simulink model "X001_AL5D_Assemby_RR_013"  (R2016a)
settings: Solver=VariableStepAuto  StartTime=0.0  StopTime=2  RelTol=1e-3
model workspace: external: MATLAB File C:\Users\Home\Google Drive\Engineering Design\Year 4 - Specialisations\Design Project 4 - Systems for Independent Living\Content\MZ\Active_Documents\AL5D Multibody Simulations\X001_AL5D_Assemby_RR_DataFile.m (data not in the file)
values from neighbouring files (symbols this model uses):
  CA = 45    [AL5D_Dataset_Creator.m]
  CAr = degtorad(CA)    [AL5D_Dataset_Creator.m]
  CFTR = CFT+(CFT*perc_disc*normrnd(0,0.5))    [AL5D_Dataset_Creator.m]
  DC = 0.09    [AL5D_Dataset_Creator.m]
  disturbance_time = 0.5    [AL5D_Dataset_Creator.m]
  disturbance_torque = disturbance_torque_array(t)    [AL5D_Dataset_Creator.m]
  DST = 0.2    [AL5D_Dataset_Creator.m]
  first_ref = first_ref_array(f)    [AL5D_Dataset_Creator.m]
  L_0 = l1+l2    (= 0.46066)    [AL5D_Dataset_Creator.m]
  RV1 = 6*2    (= 12)    [AL5D_Dataset_Creator.m]
  SC = (MM*AA)/ML    (= 50)    [AL5D_Dataset_Creator.m]
  second_ref = 0    [AL5D_Dataset_Creator.m]
  second_ref_time = 0    [AL5D_Dataset_Creator.m]
  Ts = 0.0005    [AL5D_Dataset_Creator.m]
  VS = radtodeg(1)    [AL5D_Dataset_Creator.m]
undefined symbols (not defined in the file or in its folder): smiData, X, Y, Z
libraries: sm_lib x33, fl_lib x21, nesl_utility x17, elec_lib x3, dspsrcs4 x2, simulink x1
(part 1 of 2)
settings Model: Creator=Home  LastModifiedBy=Home
settings GRTTargetCC: GeneratePreprocessorConditionals=Use local settings

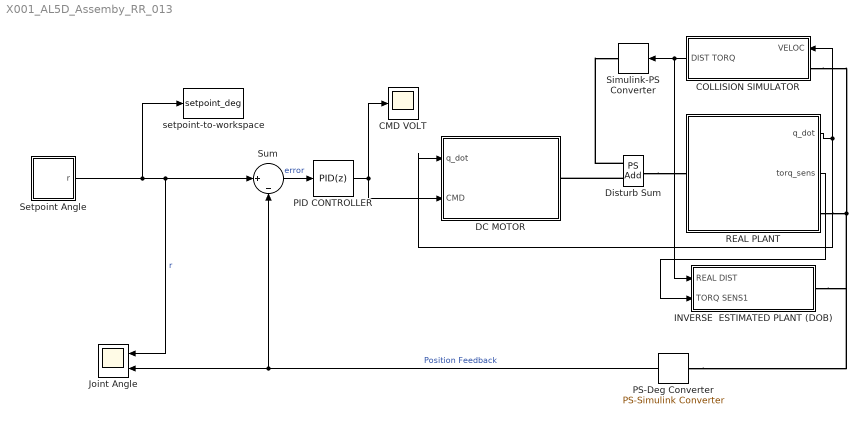
== system X001_AL5D_Assemby_RR_013 ==
  CMD VOLT : Scope
  COLLISION SIMULATOR : Subsystem
  DC MOTOR : Subsystem
  Disturb Sum : fl_lib/Physical Signals/Functions/PS Add
  INVERSE  ESTIMATED PLANT (DOB) : Subsystem
  Joint Angle : Scope  NumInputPorts=2
  PID CONTROLLER : simulink/Continuous/PID Controller  Controller=PID  TimeDomain=Discrete-time  SampleTime=Ts  IntegratorMethod=Forward Euler  FilterMethod=Forward Euler  Form=Parallel  UseFilter=on  ControllerParametersSource=internal  P=8.56066056005533  I=73.9193110956432  D=0.0561082509570558  N=2357.56103079076  InitialConditionSource=internal  InitialConditionForIntegrator=0  InitialConditionForFilter=0  ExternalReset=none  LimitOutput=on  UpperSaturationLimit=RV1  LowerSaturationLimit=-RV1  LinearizeAsGain=off  AntiWindupMode=clamping  Kb=1  TrackingMode=off  Kt=1  PParamMin=[]  PParamMax=[]  IParamMin=[]  IParamMax=[]  DParamMin=[]  DParamMax=[]  NParamMin=[]  NParamMax=[]  KbParamMin=[]  KbParamMax=[]  KtParamMin=[]  KtParamMax=[]  POutMin=[]  POutMax=[]  IOutMin=[]  IOutMax=[]  DOutMin=[]  DOutMax=[]  NOutMin=[]  NOutMax=[]  KbOutMin=[]  KbOutMax=[]  KtOutMin=[]  KtOutMax=[]  IntegratorOutMin=[]  IntegratorOutMax=[]  FilterOutMin=[]  FilterOutMax=[]  SumOutMin=[]  SumOutMax=[]  SumI1OutMin=[]  SumI1OutMax=[]  SumI2OutMin=[]  SumI2OutMax=[]  SumI3OutMin=[]  SumI3OutMax=[]  SumDOutMin=[]  SumDOutMax=[]  SaturationOutMin=[]  SaturationOutMax=[]  IntegratorContinuousStateAttributes=''  IntegratorStateMustResolveToSignalObject=off  IntegratorRTWStateStorageClass=Auto  FilterContinuousStateAttributes=''  FilterStateMustResolveToSignalObject=off  FilterRTWStateStorageClass=Auto  DifferentiatorICPrevScaledInput=0  DifferentiatorOutMin=[]  DifferentiatorOutMax=[]
  PS-Deg Converter : nesl_utility/PS-Simulink Converter  PhysicalDomain=network_engine_domain  SubClassName=ps_output  LeftPortType=input  RightPortType=output  PseudoPeriodic=off  Frequencies=[]  Unit=deg  AffineConversion=off
  REAL PLANT : Subsystem
  Setpoint Angle : Subsystem
  Simulink-PS Converter : nesl_utility/Simulink-PS Converter  PhysicalDomain=network_engine_domain  SubClassName=ps_input  LeftPortType=input  RightPortType=output  PseudoPeriodic=off  Frequencies=[]  NoiseDistribution=none  NoiseParameters=[]  Unit=N*m  AffineConversion=off  InputFiltering=off  SimscapeFilterOrder=1  InputFilterTimeConstant=0.001  UdotUserProvided=1
  Sum : Sum  Inputs=||+|-
  setpoint-to-workspace : ToWorkspace  VariableName=setpoint_deg  SaveFormat=Structure With Time  SampleTime=-1
  wires:
  PID CONTROLLER/1 -> DC MOTOR/2("CMD "), CMD VOLT/1
  Sum/1 -> PID CONTROLLER/1  "error"
  PS-Deg Converter/1 -> Sum/2, Joint Angle/2  "Position Feedback"
  REAL PLANT/1(q_dot) -> DC MOTOR/1(q_dot), COLLISION SIMULATOR/1(VELOC)
  COLLISION SIMULATOR/1(DIST TORQ) -> INVERSE  ESTIMATED PLANT (DOB)/1(REAL DIST), Simulink-PS Converter/1
  Setpoint Angle/1(r) -> setpoint-to-workspace/1, Sum/1, Joint Angle/1  "r"
  REAL PLANT/2(torq_sens) -> INVERSE  ESTIMATED PLANT (DOB)/2(TORQ SENS1)
  connections:
  Disturb Sum/LConn2 -- DC MOTOR/RConn1
  Disturb Sum/RConn1 -- REAL PLANT/LConn1
  REAL PLANT/RConn1 -- PS-Deg Converter/LConn1 -- INVERSE  ESTIMATED PLANT (DOB)/RConn1 -- COLLISION SIMULATOR/LConn1
  Disturb Sum/LConn1 -- Simulink-PS Converter/RConn1

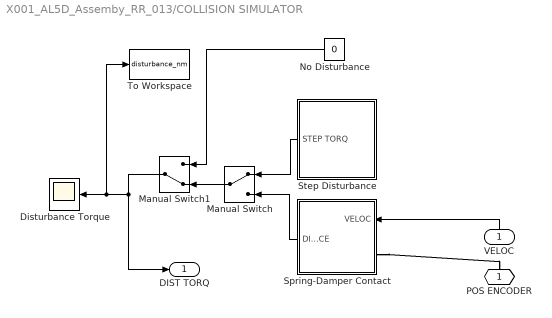
== system X001_AL5D_Assemby_RR_013/COLLISION SIMULATOR ==
  VELOC : Inport
  Disturbance Torque : Scope
  Manual Switch : ManualSwitch
  Manual Switch1 : ManualSwitch  CurrentSetting=0
  No Disturbance : Constant  Value=0
  Spring-Damper Contact : Subsystem
  Step Disturbance : Subsystem
  To Workspace : ToWorkspace  VariableName=disturbance_nm  SaveFormat=Structure With Time  SampleTime=-1
  POS ENCODER : PMIOPort  Port=1  Side=Left
  DIST TORQ : Outport
  wires:
  VELOC/1 -> Spring-Damper Contact/1(VELOC)
  Spring-Damper Contact/1(DISTURBANCE) -> Manual Switch/2
  Step Disturbance/1(STEP TORQ) -> Manual Switch/1
  Manual Switch/1 -> Manual Switch1/2
  No Disturbance/1 -> Manual Switch1/1
  Manual Switch1/1 -> To Workspace/1, Disturbance Torque/1, DIST TORQ/1
  connections:
  Spring-Damper Contact/LConn1 -- POS ENCODER/RConn1

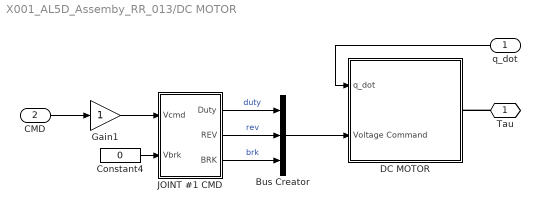
== system X001_AL5D_Assemby_RR_013/DC MOTOR ==
  q_dot : Inport
  "CMD " : Inport  Port=2
  Bus Creator : BusCreator  Inputs=3
  Constant4 : Constant  Value=0  SampleTime=Ts
  DC MOTOR : Subsystem
  Gain1 : Gain
  JOINT #1 CMD : Subsystem
  Tau : PMIOPort  Port=1  Side=Right
  wires:
  JOINT #1 CMD/1(Duty) -> Bus Creator/1  "duty"
  JOINT #1 CMD/2(REV) -> Bus Creator/2  "rev"
  Bus Creator/1 -> DC MOTOR/2(Voltage Command)
  Gain1/1 -> JOINT #1 CMD/1(Vcmd)
  JOINT #1 CMD/3(BRK) -> Bus Creator/3  "brk"
  Constant4/1 -> JOINT #1 CMD/2(Vbrk)
  "CMD "/1 -> Gain1/1
  q_dot/1 -> DC MOTOR/1(q_dot)
  connections:
  Tau/RConn1 -- DC MOTOR/RConn1

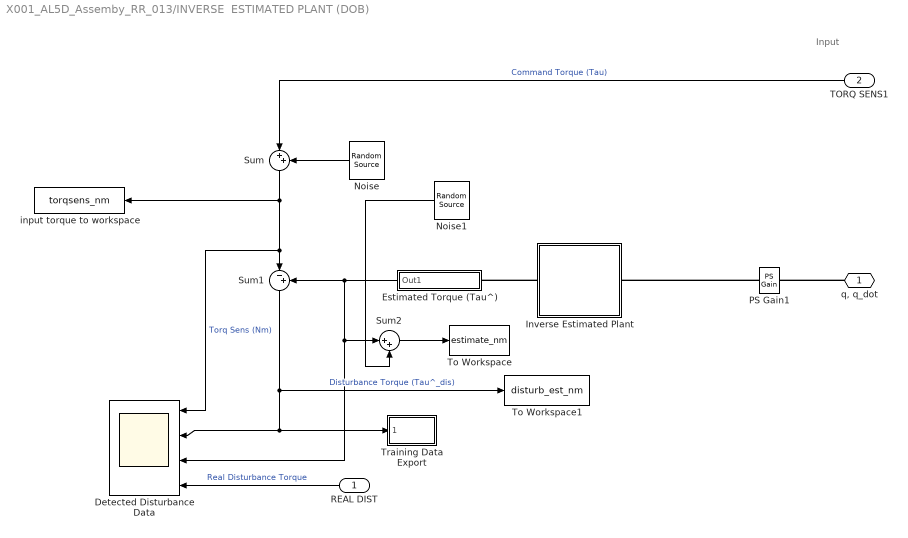
== system X001_AL5D_Assemby_RR_013/INVERSE  ESTIMATED PLANT (DOB) ==
  note: Input
  REAL DIST : Inport
  TORQ SENS1 : Inport  Port=2
  Detected Disturbance Data : Scope  NumInputPorts=4
  Estimated Torque (Tau^) : Subsystem
  Inverse Estimated Plant : Subsystem
  Noise : dspsrcs4/Random Source  SrcType=Uniform  NormMethod=Ziggurat  CltLength=12  MinVal=0  MaxVal=0.1  MeanVal=0  VarVal=1  RepMode=Not repeatable  rawSeed=1  IsInherit=off  SampMode=Discrete  SampTime=Ts*5  SampFrame=1  DataType=Double  OutComplex=Real  OutputFrames=off
  Noise1 : dspsrcs4/Random Source  SrcType=Uniform  NormMethod=Ziggurat  CltLength=12  MinVal=0  MaxVal=0.1  MeanVal=0  VarVal=1  RepMode=Not repeatable  rawSeed=1  IsInherit=off  SampMode=Discrete  SampTime=Ts*5  SampFrame=1  DataType=Double  OutComplex=Real  OutputFrames=off
  PS Gain1 : fl_lib/Physical Signals/Functions/PS Gain  gain=-1
  Sum : Sum  Inputs=|++
  Sum1 : Sum  Inputs=|-+
  Sum2 : Sum  Inputs=|++
  To Workspace : ToWorkspace  VariableName=estimate_nm  SaveFormat=Structure With Time  SampleTime=-1
  To Workspace1 : ToWorkspace  VariableName=disturb_est_nm  SaveFormat=Structure With Time  SampleTime=-1
  Training Data Export : Subsystem
  "input torque to workspace " : ToWorkspace  VariableName=torqsens_nm  SaveFormat=Structure With Time  SampleTime=-1
  "q, q_dot" : PMIOPort  Port=1  Side=Right
  wires:
  REAL DIST/1 -> Detected Disturbance Data/4  "Real Disturbance Torque"
  Sum1/1 -> To Workspace1/1, Detected Disturbance Data/2, Training Data Export/1(tau^_in)  "Disturbance Torque (Tau^_dis)"
  Estimated Torque (Tau^)/1(Out1) -> Sum2/1, Detected Disturbance Data/3, Sum1/2
  Sum/1 -> Detected Disturbance Data/1, Sum1/1, "input torque to workspace "/1  "Torq Sens (Nm)"
  TORQ SENS1/1 -> Sum/1  "Command Torque (Tau)"
  Noise/1 -> Sum/2
  Noise1/1 -> Sum2/2
  Sum2/1 -> To Workspace/1
  connections:
  Inverse Estimated Plant/RConn1 -- Estimated Torque (Tau^)/LConn1
  "q, q_dot"/RConn1 -- PS Gain1/LConn1
  PS Gain1/RConn1 -- Inverse Estimated Plant/LConn1

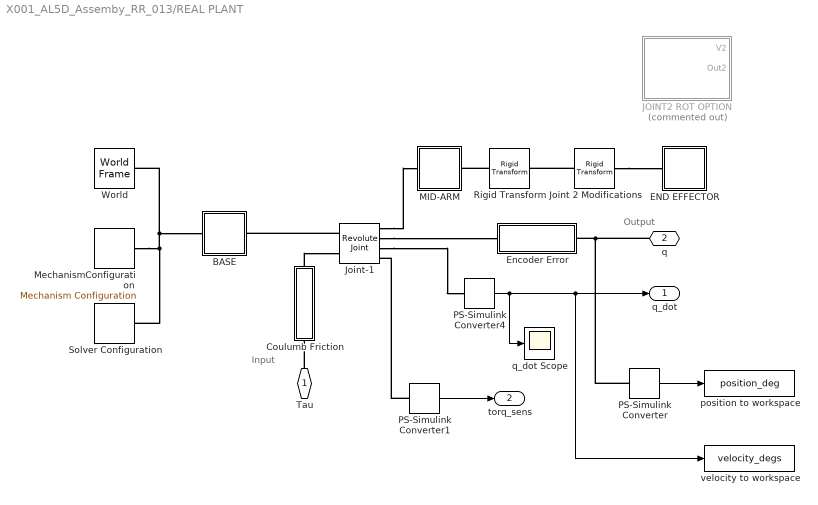
== system X001_AL5D_Assemby_RR_013/REAL PLANT ==
  note: Output
  note: Input
  BASE : Subsystem
  Coulumb Friction : Subsystem
  END EFFECTOR : Subsystem
  Encoder Error : Subsystem
  JOINT2 ROT OPTION : Subsystem  Commented=on
  Joint 2 Modifications : sm_lib/Frames and Transforms/Rigid Transform  TranslationMethod=None  TranslationLengthUnit=m  TranslationStandardAxis=+Z  TranslationStandardOffset=0  TranslationCartesianOffset=[0 0 0]  TranslationROffset=0  TranslationROffsetUnits=m  TranslationZOffset=0  TranslationZOffsetUnits=m  TranslationThetaOffset=0  TranslationThetaOffsetUnits=deg  RotationMethod=StandardAxis  RotationAngleUnits=deg  RotationStandardAxis=+Z  RotationAngle=0  RotationArbitraryAxis=[0 0 1]  FollAlignAxisA=+X  BaseAlignAxisA=+Y  FollAlignAxisB=+Y  BaseAlignAxisB=+Z  RotationSequenceAxes=FollowerAxes  RotationSequence=XYX  RotationSequenceAngles=[0 0 0]  RotationSequenceAnglesUnits=deg  RotationMatrix=[1 0 0; 0 1 0; 0 0 1]
  Joint-1 : sm_lib/Joints/Revolute Joint  SenseConstraintForce=off  SenseConstraintForceX=off  SenseConstraintForceY=off  SenseConstraintForceZ=off  SenseConstraintTorque=off  SenseConstraintTorqueX=off  SenseConstraintTorqueY=off  SenseConstraintTorqueZ=off  SenseTotalForce=off  SenseTotalForceX=off  SenseTotalForceY=off  SenseTotalForceZ=off  SenseTotalTorque=off  SenseTotalTorqueX=off  SenseTotalTorqueY=off  SenseTotalTorqueZ=off  CompositeWrenchDir=FollowerOnBase  CompositeWrenchFrame=BaseFrame  EquilibriumPosition=0  EquilibriumPositionUnits=rad  SpringStiffness=JSSR  SpringStiffnessUnits=m*N/rad  DampingCoefficient=JDCR  DampingCoefficientUnits=m*s*N/rad  TorqueActuationMode=InputTorque  MotionActuationMode=ComputedMotion  SensePosition=on  SenseVelocity=on  SenseAcceleration=off  SenseTorqueForce=on  PositionTargetSpecify=off  PositionTargetPriority=Low  PositionTargetValue=-90  PositionTargetValueUnits=deg  VelocityTargetSpecify=off  VelocityTargetPriority=High  VelocityTargetValue=-30  VelocityTargetValueUnits=deg/s
  MID-ARM : Subsystem
  MechanismConfiguration : sm_lib/Utilities/Mechanism Configuration  UniformGravity=Constant  GravityVector=[0 0 -9.81]  GravityUnits=m/s^2  LinearizationDelta=0.001
  PS-Simulink Converter : nesl_utility/PS-Simulink Converter  PhysicalDomain=network_engine_domain  SubClassName=ps_output  LeftPortType=input  RightPortType=output  PseudoPeriodic=off  Frequencies=[]  Unit=deg  AffineConversion=off
  PS-Simulink Converter1 : nesl_utility/PS-Simulink Converter  PhysicalDomain=network_engine_domain  SubClassName=ps_output  LeftPortType=input  RightPortType=output  PseudoPeriodic=off  Frequencies=[]  Unit=N*m  AffineConversion=off
  PS-Simulink Converter4 : nesl_utility/PS-Simulink Converter  PhysicalDomain=network_engine_domain  SubClassName=ps_output  LeftPortType=input  RightPortType=output  PseudoPeriodic=off  Frequencies=[]  Unit=deg/s  AffineConversion=off
  Rigid Transform : sm_lib/Frames and Transforms/Rigid Transform  TranslationMethod=None  TranslationLengthUnit=m  TranslationStandardAxis=+Z  TranslationStandardOffset=0  TranslationCartesianOffset=[0 0 0]  TranslationROffset=0  TranslationROffsetUnits=m  TranslationZOffset=0  TranslationZOffsetUnits=m  TranslationThetaOffset=0  TranslationThetaOffsetUnits=deg  RotationMethod=ArbitraryAxis  RotationAngleUnits=deg  RotationStandardAxis=+Z  RotationAngle=-90  RotationArbitraryAxis=[0 0 1]  FollAlignAxisA=+X  BaseAlignAxisA=+Y  FollAlignAxisB=+Y  BaseAlignAxisB=+Z  RotationSequenceAxes=FollowerAxes  RotationSequence=XYX  RotationSequenceAngles=[0 0 0]  RotationSequenceAnglesUnits=deg  RotationMatrix=[1 0 0; 0 1 0; 0 0 1]
  Solver Configuration : nesl_utility/Solver Configuration  PhysicalDomain=network_engine_domain  SubClassName=solver  LeftPortType=input  RightPortType=generic  Accelerate=off  Tones=[]  Harmonics=[]  SimulateNoise=off  Profile=off  UseLocalSampling=off  EnableSwitchedLinearOptims=on  FrequencyDomain=off  UseCCode=off  RelTol=0.001  AbsTol=1e-06  MinStep=1e-09  ToWorkspace=off  RevertToSquareIcSolve=off  NumHomotopyIterations=100  PhasorMode=off  PhasorModeNumHarmonics=1  OverrideAbsTol=off  DoDC=off  ResidualTolerance=1e-09  UseLocalSolver=off  LocalSolverChoice=NE_BACKWARD_EULER_ADVANCER  LocalSolverSampleTime=0.001  DoFixedCost=off  MaxNonlinIter=3  MaxModeIter=2  LinearAlgebra=Sparse  DelaysMemoryBudget=1024  AutomaticFiltering=on  FilteringTimeConstant=0.001
  World : sm_lib/Frames and Transforms/World Frame
  position to workspace : ToWorkspace  VariableName=position_deg  SaveFormat=Structure With Time  SampleTime=-1
  q_dot Scope : Scope
  velocity to workspace : ToWorkspace  VariableName=velocity_degs  SaveFormat=Structure With Time  SampleTime=-1
  Tau : PMIOPort  Port=1  Side=Left
  q : PMIOPort  Port=2  Side=Right
  q_dot : Outport
  torq_sens : Outport  Port=2
  wires:
  PS-Simulink Converter/1 -> position to workspace/1
  PS-Simulink Converter4/1 -> velocity to workspace/1, q_dot/1, q_dot Scope/1
  PS-Simulink Converter1/1 -> torq_sens/1
  connections:
  World/RConn1 -- MechanismConfiguration/RConn1 -- Solver Configuration/RConn1 -- BASE/LConn1
  Rigid Transform/LConn1 -- MID-ARM/RConn1
  Joint-1/RConn3 -- PS-Simulink Converter4/LConn1
  Joint-1/LConn1 -- BASE/RConn1
  Joint-1/RConn1 -- MID-ARM/LConn1
  Joint 2 Modifications/RConn1 -- END EFFECTOR/RConn1
  PS-Simulink Converter1/LConn1 -- Joint-1/RConn4
  Joint 2 Modifications/LConn1 -- Rigid Transform/RConn1
  Joint-1/RConn2 -- Encoder Error/LConn1
  Coulumb Friction/RConn1 -- Joint-1/LConn2
  Tau/RConn1 -- Coulumb Friction/LConn1
  q/RConn1 -- PS-Simulink Converter/LConn1 -- Encoder Error/RConn1

== system X001_AL5D_Assemby_RR_013/Setpoint Angle ==
  Setpoint Angle : Step  Time=0  After=first_ref  SampleTime=0
  Setpoint Angle1 : Step  Commented=on  Time=second_ref_time  After=second_ref  SampleTime=0
  Sum1 : Sum  Inputs=|++
  r : Outport
  wires:
  Sum1/1 -> r/1
  Setpoint Angle/1 -> Sum1/1  "REF1"
  Setpoint Angle1/1 -> Sum1/2

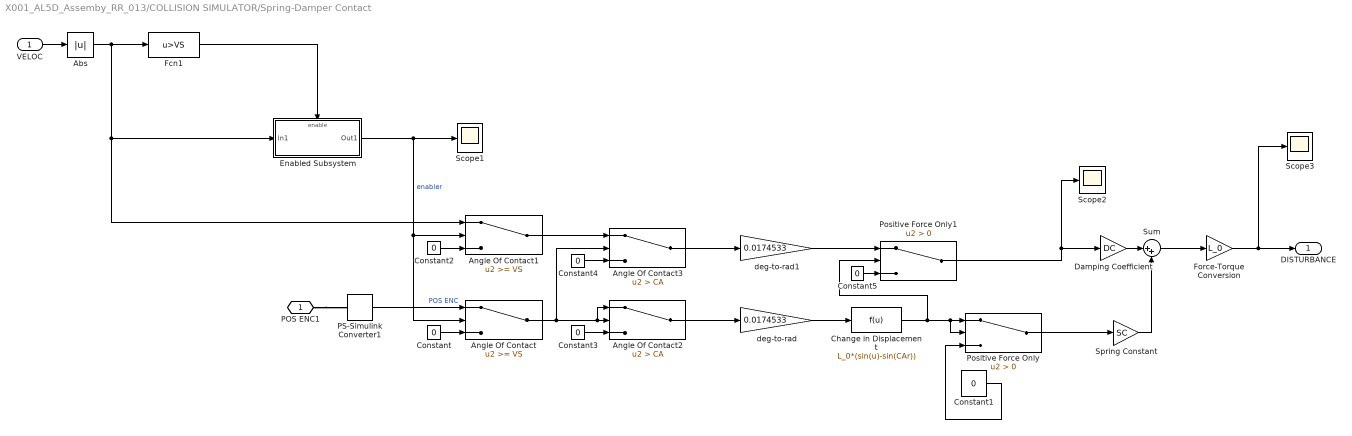
== system X001_AL5D_Assemby_RR_013/COLLISION SIMULATOR/Spring-Damper Contact ==
  VELOC : Inport
  Abs : Abs
  Angle Of Contact : Switch  Threshold=VS
  Angle Of Contact1 : Switch  Threshold=VS
  Angle Of Contact2 : Switch  Criteria=u2 > Threshold  Threshold=CA
  Angle Of Contact3 : Switch  Criteria=u2 > Threshold  Threshold=CA
  Change in Displacement : Fcn  Expr=L_0*(sin(u)-sin(CAr))
  Constant{,1..5} (6 alike) : Constant  Value=0
  Damping Coefficient : Gain  Gain=DC
  Enabled Subsystem : Subsystem  TreatAsAtomicUnit=on
  Fcn1 : Fcn  Expr=u>VS
  Force-Torque Conversion : Gain  Gain=L_0
  PS-Simulink Converter1 : nesl_utility/PS-Simulink Converter  PhysicalDomain=network_engine_domain  SubClassName=ps_output  LeftPortType=input  RightPortType=output  PseudoPeriodic=off  Frequencies=[]  Unit=deg  AffineConversion=off
  Positive Force Only : Switch  Criteria=u2 > Threshold
  Positive Force Only1 : Switch  Criteria=u2 > Threshold
  Scope1 : Scope
  Scope2 : Scope
  Scope3 : Scope
  Spring Constant : Gain  Gain=SC
  Sum : Sum  Inputs=|++
  deg-to-rad : Gain  Gain=0.0174533
  deg-to-rad1 : Gain  Gain=0.0174533
  POS ENC1 : PMIOPort  Port=1  Side=Left
  DISTURBANCE : Outport
  wires:
  Sum/1 -> Force-Torque Conversion/1
  PS-Simulink Converter1/1 -> Angle Of Contact/1  "POS ENC"
  Change in Displacement/1 -> Positive Force Only1/2, Positive Force Only/2, Positive Force Only/1
  Constant/1 -> Angle Of Contact/3
  Spring Constant/1 -> Sum/2
  Positive Force Only/1 -> Spring Constant/1
  Constant1/1 -> Positive Force Only/3
  Angle Of Contact/1 -> Angle Of Contact3/2, Angle Of Contact2/2, Angle Of Contact2/1
  Angle Of Contact1/1 -> Angle Of Contact3/1
  deg-to-rad/1 -> Change in Displacement/1
  Constant2/1 -> Angle Of Contact1/3
  Damping Coefficient/1 -> Sum/1
  deg-to-rad1/1 -> Positive Force Only1/1
  Positive Force Only1/1 -> Scope2/1, Damping Coefficient/1
  Constant3/1 -> Angle Of Contact2/3
  Constant4/1 -> Angle Of Contact3/3
  Angle Of Contact2/1 -> deg-to-rad/1
  Angle Of Contact3/1 -> deg-to-rad1/1
  VELOC/1 -> Abs/1
  Abs/1 -> Fcn1/1, Angle Of Contact1/1, Enabled Subsystem/1(In1)
  Fcn1/1 -> Enabled Subsystem/Enable
  Enabled Subsystem/1(Out1) -> Angle Of Contact/2, Angle Of Contact1/2, Scope1/1  "enabler"
  Force-Torque Conversion/1 -> Scope3/1, DISTURBANCE/1
  Constant5/1 -> Positive Force Only1/3
  connections:
  POS ENC1/RConn1 -- PS-Simulink Converter1/LConn1

== system X001_AL5D_Assemby_RR_013/COLLISION SIMULATOR/Step Disturbance ==
  Step : Step  Time=disturbance_time  After=disturbance_torque  SampleTime=0
  Step1 : Step  Time=disturbance_time+0.2  After=-disturbance_torque  SampleTime=0
  Sum1 : Sum  Inputs=|++
  STEP TORQ : Outport
  wires:
  Step/1 -> Sum1/1
  Step1/1 -> Sum1/2
  Sum1/1 -> STEP TORQ/1

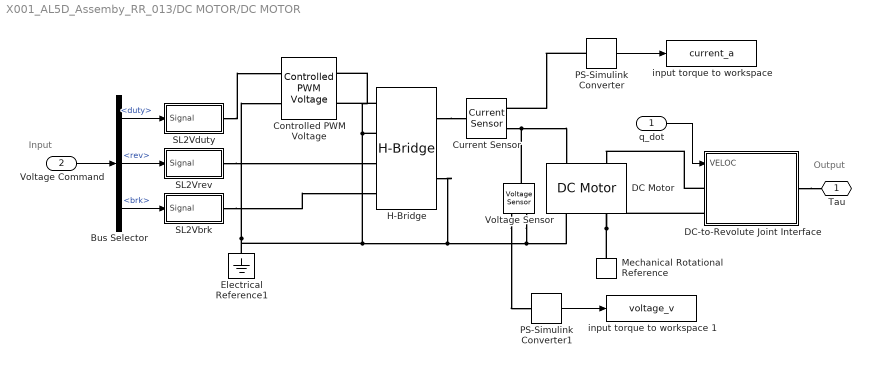
== system X001_AL5D_Assemby_RR_013/DC MOTOR/DC MOTOR ==
  note: Input
  note: Output
  q_dot : Inport
  Voltage Command : Inport  Port=2
  Bus Selector : BusSelector  OutputSignals=duty,rev,brk
  Controlled PWM Voltage : elec_lib/Actuators & Drivers/Drivers/Controlled PWM Voltage  F=400 Hz  TD=0 s  pulse_width_offset=0 s  Vmin=0 V  Vmax=RV1 V  Vm=RV1 V  pwm_or_av=2  event_type=1  sample_time=1e-6 s
  Current Sensor : fl_lib/Electrical/Electrical Sensors/Current Sensor
  DC Motor : elec_lib/Actuators & Drivers/Rotational Actuators/DC Motor  parameterization=2  Ra=3.9 Ohm  La=L1 H  emf_or_torque=1  Kv=7.2e-5 V/rpm  Ki=6.876e-4 N*m/A  T_stall=ST1 N*m  w_max=NLS1 rpm  w_rated=1.5e+4 rpm  P_rated=0.08 W  V_rated=RV1 V  J=0.01 g*cm^2  lam_param=2  lam=0 N*m/(rad/s)  i_noload=NLC1 A  V_i_noload=RV1 V  speed0=0 rpm  alpha=0.00393 1/K  Tmeas=25 degC  thermal_mass=100 J/K  initial_temperature=25 degC
  DC-to-Revolute Joint Interface : Subsystem
  Electrical Reference1 : fl_lib/Electrical/Electrical Elements/Electrical Reference
  H-Bridge : elec_lib/Actuators & Drivers/Drivers/H-Bridge  Venable=2.5 V  Vmax=RV1 V  Vreverse=2.5 V  Vbrake=2.5 V  Vm=RV1 V  pwm_or_av=2  discontinuous=0  freewheeling_mode=1  freewheeling_mode_disc=1  Ron=0.1 Ohm  Don=0.05 Ohm  Rload=10 Ohm  Lload=1e-5 H  F=10 kHz  thermal_mass=100 J/K  initial_temperature=298.15 K  Ron2=0.1 Ohm  Don2=0.05 Ohm  Tmeas=298.15 K  Tmeas2=398.15 K
  Mechanical Rotational Reference : fl_lib/Mechanical/Rotational Elements/Mechanical Rotational Reference
  PS-Simulink Converter : nesl_utility/PS-Simulink Converter  PhysicalDomain=network_engine_domain  SubClassName=ps_output  LeftPortType=input  RightPortType=output  PseudoPeriodic=off  Frequencies=[]  Unit=A  AffineConversion=off
  PS-Simulink Converter1 : nesl_utility/PS-Simulink Converter  PhysicalDomain=network_engine_domain  SubClassName=ps_output  LeftPortType=input  RightPortType=output  PseudoPeriodic=off  Frequencies=[]  Unit=V  AffineConversion=off
  SL2Vbrk : Subsystem
  SL2Vduty : Subsystem
  SL2Vrev : Subsystem
  Voltage Sensor : fl_lib/Electrical/Electrical Sensors/Voltage Sensor
  "input torque to workspace " : ToWorkspace  VariableName=current_a  SaveFormat=Structure With Time  SampleTime=-1
  input torque to workspace 1 : ToWorkspace  VariableName=voltage_v  SaveFormat=Structure With Time  SampleTime=-1
  Tau : PMIOPort  Port=1  Side=Right
  wires:
  q_dot/1 -> DC-to-Revolute Joint Interface/1(VELOC)
  Bus Selector/1 -> SL2Vduty/1(Signal)  "<duty>"
  Bus Selector/2 -> SL2Vrev/1(Signal)  "<rev>"
  Bus Selector/3 -> SL2Vbrk/1(Signal)  "<brk>"
  Voltage Command/1 -> Bus Selector/1
  PS-Simulink Converter/1 -> "input torque to workspace "/1
  PS-Simulink Converter1/1 -> input torque to workspace 1/1
  connections:
  H-Bridge/LConn2 -- Electrical Reference1/LConn1 -- Controlled PWM Voltage/LConn2 -- Voltage Sensor/RConn2 -- DC Motor/RConn1 -- H-Bridge/RConn2 -- Controlled PWM Voltage/RConn2
  DC-to-Revolute Joint Interface/LConn1 -- DC Motor/LConn2
  DC-to-Revolute Joint Interface/LConn2 -- Mechanical Rotational Reference/LConn1 -- DC Motor/RConn2
  SL2Vrev/RConn1 -- H-Bridge/LConn3
  SL2Vduty/RConn1 -- Controlled PWM Voltage/LConn1
  H-Bridge/LConn1 -- Controlled PWM Voltage/RConn1
  SL2Vbrk/RConn1 -- H-Bridge/LConn4
  DC-to-Revolute Joint Interface/RConn1 -- Tau/RConn1
  H-Bridge/RConn1 -- Current Sensor/LConn1
  Current Sensor/RConn2 -- Voltage Sensor/LConn1 -- DC Motor/LConn1
  PS-Simulink Converter/LConn1 -- Current Sensor/RConn1
  Voltage Sensor/RConn1 -- PS-Simulink Converter1/LConn1

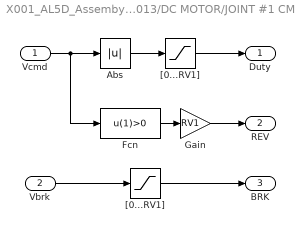
== system X001_AL5D_Assemby_RR_013/DC MOTOR/JOINT #1 CMD ==
  Vcmd : Inport
  Vbrk : Inport  Port=2
  Abs : Abs
  Fcn : Fcn  Expr=u(1)>0
  Gain : Gain  Gain=RV1
  "[0...RV1]" : Saturate  UpperLimit=RV1  LowerLimit=0
  "[0...RV1] " : Saturate  UpperLimit=RV1  LowerLimit=0
  Duty : Outport
  REV : Outport  Port=2
  BRK : Outport  Port=3
  wires:
  "[0...RV1] "/1 -> BRK/1
  Vbrk/1 -> "[0...RV1] "/1
  Vcmd/1 -> Fcn/1, Abs/1
  Abs/1 -> "[0...RV1]"/1
  Fcn/1 -> Gain/1
  "[0...RV1]"/1 -> Duty/1
  Gain/1 -> REV/1

== system X001_AL5D_Assemby_RR_013/INVERSE  ESTIMATED PLANT (DOB)/Estimated Torque (Tau^) ==
  PS Add : fl_lib/Physical Signals/Functions/PS Add
  PS Constant : fl_lib/Physical Signals/Sources/PS Constant  constant=CFT
  PS-Simulink Converter : nesl_utility/PS-Simulink Converter  PhysicalDomain=network_engine_domain  SubClassName=ps_output  LeftPortType=input  RightPortType=output  PseudoPeriodic=off  Frequencies=[]  Unit=N*m  AffineConversion=off
  Conn1 : PMIOPort  Port=1  Side=Left
  Out1 : Outport
  wires:
  PS-Simulink Converter/1 -> Out1/1  "Estimated Torque (Tau^)"
  connections:
  PS Constant/RConn1 -- PS Add/LConn1
  Conn1/RConn1 -- PS Add/LConn2
  PS Add/RConn1 -- PS-Simulink Converter/LConn1

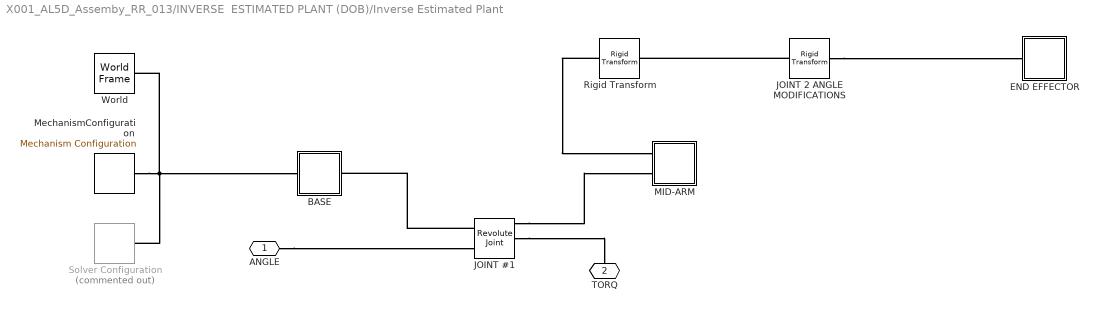
== system X001_AL5D_Assemby_RR_013/INVERSE  ESTIMATED PLANT (DOB)/Inverse Estimated Plant ==
  BASE : Subsystem
  END EFFECTOR : Subsystem
  JOINT #1 : sm_lib/Joints/Revolute Joint  SenseConstraintForce=off  SenseConstraintForceX=off  SenseConstraintForceY=off  SenseConstraintForceZ=off  SenseConstraintTorque=off  SenseConstraintTorqueX=off  SenseConstraintTorqueY=off  SenseConstraintTorqueZ=off  SenseTotalForce=off  SenseTotalForceX=off  SenseTotalForceY=off  SenseTotalForceZ=off  SenseTotalTorque=on  SenseTotalTorqueX=off  SenseTotalTorqueY=off  SenseTotalTorqueZ=off  CompositeWrenchDir=FollowerOnBase  CompositeWrenchFrame=BaseFrame  EquilibriumPosition=0  EquilibriumPositionUnits=rad  SpringStiffness=JSS  SpringStiffnessUnits=m*N/rad  DampingCoefficient=JDC  DampingCoefficientUnits=m*s*N/rad  TorqueActuationMode=ComputedTorque  MotionActuationMode=InputMotion  SensePosition=off  SenseVelocity=off  SenseAcceleration=off  SenseTorqueForce=on  PositionTargetSpecify=off  PositionTargetPriority=Low  PositionTargetValue=-90  PositionTargetValueUnits=deg  VelocityTargetSpecify=off  VelocityTargetPriority=High  VelocityTargetValue=-30  VelocityTargetValueUnits=deg/s
  JOINT 2 ANGLE MODIFICATIONS : sm_lib/Frames and Transforms/Rigid Transform  TranslationMethod=None  TranslationLengthUnit=m  TranslationStandardAxis=+Z  TranslationStandardOffset=0  TranslationCartesianOffset=[0 0 0]  TranslationROffset=0  TranslationROffsetUnits=m  TranslationZOffset=0  TranslationZOffsetUnits=m  TranslationThetaOffset=0  TranslationThetaOffsetUnits=deg  RotationMethod=StandardAxis  RotationAngleUnits=deg  RotationStandardAxis=+Z  RotationAngle=0  RotationArbitraryAxis=[0 0 1]  FollAlignAxisA=+X  BaseAlignAxisA=+Y  FollAlignAxisB=+Y  BaseAlignAxisB=+Z  RotationSequenceAxes=FollowerAxes  RotationSequence=XYX  RotationSequenceAngles=[0 0 0]  RotationSequenceAnglesUnits=deg  RotationMatrix=[1 0 0; 0 1 0; 0 0 1]
  MID-ARM : Subsystem
  MechanismConfiguration : sm_lib/Utilities/Mechanism Configuration  UniformGravity=Constant  GravityVector=[0 0 -9.81]  GravityUnits=m/s^2  LinearizationDelta=0.001
  Rigid Transform : sm_lib/Frames and Transforms/Rigid Transform  TranslationMethod=None  TranslationLengthUnit=m  TranslationStandardAxis=+Z  TranslationStandardOffset=0  TranslationCartesianOffset=[0 0 0]  TranslationROffset=0  TranslationROffsetUnits=m  TranslationZOffset=0  TranslationZOffsetUnits=m  TranslationThetaOffset=0  TranslationThetaOffsetUnits=deg  RotationMethod=ArbitraryAxis  RotationAngleUnits=deg  RotationStandardAxis=+Z  RotationAngle=-90  RotationArbitraryAxis=[0 0 1]  FollAlignAxisA=+X  BaseAlignAxisA=+Y  FollAlignAxisB=+Y  BaseAlignAxisB=+Z  RotationSequenceAxes=FollowerAxes  RotationSequence=XYX  RotationSequenceAngles=[0 0 0]  RotationSequenceAnglesUnits=deg  RotationMatrix=[1 0 0; 0 1 0; 0 0 1]
  Solver Configuration : nesl_utility/Solver Configuration  Commented=on  PhysicalDomain=network_engine_domain  SubClassName=solver  LeftPortType=input  RightPortType=generic  Accelerate=off  Tones=[]  Harmonics=[]  SimulateNoise=off  Profile=off  UseLocalSampling=off  EnableSwitchedLinearOptims=on  FrequencyDomain=off  UseCCode=off  RelTol=0.001  AbsTol=1e-06  MinStep=1e-09  ToWorkspace=off  RevertToSquareIcSolve=off  NumHomotopyIterations=100  PhasorMode=off  PhasorModeNumHarmonics=1  OverrideAbsTol=off  DoDC=off  ResidualTolerance=1e-09  UseLocalSolver=off  LocalSolverChoice=NE_BACKWARD_EULER_ADVANCER  LocalSolverSampleTime=0.001  DoFixedCost=off  MaxNonlinIter=3  MaxModeIter=2  LinearAlgebra=Sparse  DelaysMemoryBudget=1024  AutomaticFiltering=on  FilteringTimeConstant=0.001
  World : sm_lib/Frames and Transforms/World Frame
  ANGLE : PMIOPort  Port=1  Side=Left
  TORQ : PMIOPort  Port=2  Side=Right
  connections:
  Rigid Transform/LConn1 -- MID-ARM/LConn1
  World/RConn1 -- BASE/LConn1 -- MechanismConfiguration/RConn1 -- Solver Configuration/RConn1
  JOINT #1/RConn1 -- MID-ARM/LConn2
  JOINT #1/LConn1 -- BASE/RConn1
  ANGLE/RConn1 -- JOINT #1/LConn2
  JOINT 2 ANGLE MODIFICATIONS/LConn1 -- Rigid Transform/RConn1
  JOINT 2 ANGLE MODIFICATIONS/RConn1 -- END EFFECTOR/RConn1
  JOINT #1/RConn2 -- TORQ/RConn1

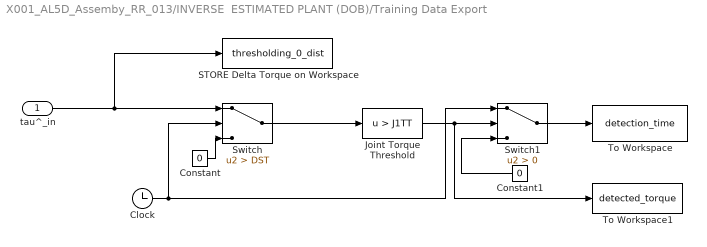
== system X001_AL5D_Assemby_RR_013/INVERSE  ESTIMATED PLANT (DOB)/Training Data Export ==
  tau^_in : Inport
  Clock : Clock
      settings: Decimation=100
  Constant : Constant  Value=0
  Constant1 : Constant  Value=0
  Joint Torque Threshold : Fcn  Expr=u > J1TT
  STORE Delta Torque on Workspace : ToWorkspace  VariableName=thresholding_0_dist  SaveFormat=Structure With Time  SampleTime=-1
  Switch : Switch  Criteria=u2 > Threshold  Threshold=DST
  Switch1 : Switch  Criteria=u2 > Threshold
  To Workspace : ToWorkspace  VariableName=detection_time  SampleTime=-1
  To Workspace1 : ToWorkspace  VariableName=detected_torque  SaveFormat=Timeseries  SampleTime=-1
  wires:
  Switch1/1 -> To Workspace/1
  Clock/1 -> Switch/2, Switch1/1
  Constant/1 -> Switch/3
  Switch/1 -> Joint Torque Threshold/1
  Joint Torque Threshold/1 -> Switch1/2, To Workspace1/1
  Constant1/1 -> Switch1/3
  tau^_in/1 -> STORE Delta Torque on Workspace/1, Switch/1

== system X001_AL5D_Assemby_RR_013/REAL PLANT/BASE ==
  ReferenceFrame : sm_lib/Frames and Transforms/Reference Frame
  Solid : sm_lib/Body Elements/Solid  InertiaType=Custom  Mass=smiData.Solid(2).mass  MassUnits=kg  CenterOfMass=smiData.Solid(2).CoM  CenterOfMassUnits=mm  MomentsOfInertia=smiData.Solid(2).MoI  MomentsOfInertiaUnits=kg*mm^2  ProductsOfInertia=smiData.Solid(2).PoI  ProductsOfInertiaUnits=kg*mm^2  DensityBased=on  Density=1000  DensityUnits=kg/(m^3)  DoExposeReferenceFrame=on  SerializedFrames=<Frames/>  GraphicType=FromGeometry  MarkerShape=Sphere  MarkerSize=10  GraphicVisPropType=SimpleVisualProperties  GraphicDiffuseColor=smiData.Solid(2).color  GraphicSpecularColor=[0.5 0.5 0.5 1.0]  GraphicAmbientColor=[0.15 0.15 0.15 1.0]  GraphicEmissiveColor=[0.0 0.0 0.0 1.0]  GraphicShininess=75  GraphicOpacity=smiData.Solid(2).opacity  GeometryShape=FromFile  RectangleSize=[1 1]  RectangleSizeUnits=m  BrickDimensions=[1 1 1]  BrickDimensionUnits=m  CylinderRadius=1  CylinderRadiusUnits=m  CylinderLength=1  CylinderLengthUnits=m  SphereRadius=1  SphereRadiusUnits=m  EllipsoidRadii=[1 1 1]  EllipsoidRadiiUnits=m  ExtrusionCrossSection=[1 1; -1 1; -1 -1; 1 -1]  ExtrusionCrossSectionUnits=m  ExtrusionLength=1  ExtrusionLengthUnits=m  PolygonNumSides=3  PolygonOuterRadius=1  PolygonOuterRadiusUnits=m  ExtGeomFileType=STEP  ExtGeomFileName=X001_AL5D_Base_Subassy_Default_sldprt.STEP  ExtGeomFileUnits=m  RevolutionCrossSection=[1 1; 1 -1; 2 -1; 2 1]  RevolutionCrossSectionUnits=m  RevolutionExtent=Full  RevolutionAngle=180  RevolutionAngleUnits=deg
  Transform : sm_lib/Frames and Transforms/Rigid Transform  TranslationMethod=Cartesian  TranslationLengthUnit=mm  TranslationStandardAxis=+Z  TranslationStandardOffset=0  TranslationCartesianOffset=smiData.RigidTransform(1).translation  TranslationROffset=0  TranslationROffsetUnits=m  TranslationZOffset=0  TranslationZOffsetUnits=m  TranslationThetaOffset=0  TranslationThetaOffsetUnits=deg  RotationMethod=ArbitraryAxis  RotationAngleUnits=rad  RotationStandardAxis=+Z  RotationAngle=smiData.RigidTransform(1).angle  RotationArbitraryAxis=smiData.RigidTransform(1).axis  FollAlignAxisA=+X  BaseAlignAxisA=+Y  FollAlignAxisB=+Y  BaseAlignAxisB=+Z  RotationSequenceAxes=FollowerAxes  RotationSequence=XYX  RotationSequenceAngles=[0 0 0]  RotationSequenceAnglesUnits=deg  RotationMatrix=[1 0 0; 0 1 0; 0 0 1]
  Transform1 : sm_lib/Frames and Transforms/Rigid Transform  TranslationMethod=Cartesian  TranslationLengthUnit=mm  TranslationStandardAxis=+Z  TranslationStandardOffset=0  TranslationCartesianOffset=smiData.RigidTransform(3).translation  TranslationROffset=0  TranslationROffsetUnits=m  TranslationZOffset=0  TranslationZOffsetUnits=m  TranslationThetaOffset=0  TranslationThetaOffsetUnits=deg  RotationMethod=ArbitraryAxis  RotationAngleUnits=rad  RotationStandardAxis=+Z  RotationAngle=smiData.RigidTransform(3).angle  RotationArbitraryAxis=smiData.RigidTransform(3).axis  FollAlignAxisA=+X  BaseAlignAxisA=+Y  FollAlignAxisB=+Y  BaseAlignAxisB=+Z  RotationSequenceAxes=FollowerAxes  RotationSequence=XYX  RotationSequenceAngles=[0 0 0]  RotationSequenceAnglesUnits=deg  RotationMatrix=[1 0 0; 0 1 0; 0 0 1]
  F : PMIOPort  Port=1  Side=Left
  F1 : PMIOPort  Port=2  Side=Right
  connections:
  Solid/RConn1 -- ReferenceFrame/RConn1 -- Transform/LConn1 -- Transform1/LConn1
  Transform/RConn1 -- F/RConn1
  F1/RConn1 -- Transform1/RConn1

== system X001_AL5D_Assemby_RR_013/REAL PLANT/Coulumb Friction ==
  Coulumb Friction : fl_lib/Physical Signals/Sources/PS Constant  constant=-CFTR
  PS Add1 : fl_lib/Physical Signals/Functions/PS Add
  Tau_out : PMIOPort  Port=1  Side=Right
  Tau_in : PMIOPort  Port=2  Side=Left
  connections:
  Coulumb Friction/RConn1 -- PS Add1/LConn2
  Tau_in/RConn1 -- PS Add1/LConn1
  PS Add1/RConn1 -- Tau_out/RConn1

== system X001_AL5D_Assemby_RR_013/REAL PLANT/END EFFECTOR ==
  ReferenceFrame : sm_lib/Frames and Transforms/Reference Frame
  Solid : sm_lib/Body Elements/Solid  InertiaType=Custom  Mass=smiData.Solid(1).mass  MassUnits=kg  CenterOfMass=smiData.Solid(1).CoM  CenterOfMassUnits=mm  MomentsOfInertia=smiData.Solid(1).MoI  MomentsOfInertiaUnits=kg*mm^2  ProductsOfInertia=smiData.Solid(1).PoI  ProductsOfInertiaUnits=kg*mm^2  DensityBased=on  Density=1000  DensityUnits=kg/(m^3)  DoExposeReferenceFrame=on  SerializedFrames=<Frames/>  GraphicType=FromGeometry  MarkerShape=Sphere  MarkerSize=10  GraphicVisPropType=SimpleVisualProperties  GraphicDiffuseColor=smiData.Solid(1).color  GraphicSpecularColor=[0.5 0.5 0.5 1.0]  GraphicAmbientColor=[0.15 0.15 0.15 1.0]  GraphicEmissiveColor=[0.0 0.0 0.0 1.0]  GraphicShininess=75  GraphicOpacity=smiData.Solid(1).opacity  GeometryShape=FromFile  RectangleSize=[1 1]  RectangleSizeUnits=m  BrickDimensions=[1 1 1]  BrickDimensionUnits=m  CylinderRadius=1  CylinderRadiusUnits=m  CylinderLength=1  CylinderLengthUnits=m  SphereRadius=1  SphereRadiusUnits=m  EllipsoidRadii=[1 1 1]  EllipsoidRadiiUnits=m  ExtrusionCrossSection=[1 1; -1 1; -1 -1; 1 -1]  ExtrusionCrossSectionUnits=m  ExtrusionLength=1  ExtrusionLengthUnits=m  PolygonNumSides=3  PolygonOuterRadius=1  PolygonOuterRadiusUnits=m  ExtGeomFileType=STEP  ExtGeomFileName=End_effector_subassy_Default_sldprt.STEP  ExtGeomFileUnits=m  RevolutionCrossSection=[1 1; 1 -1; 2 -1; 2 1]  RevolutionCrossSectionUnits=m  RevolutionExtent=Full  RevolutionAngle=180  RevolutionAngleUnits=deg
  Transform : sm_lib/Frames and Transforms/Rigid Transform  TranslationMethod=Cartesian  TranslationLengthUnit=mm  TranslationStandardAxis=+Z  TranslationStandardOffset=0  TranslationCartesianOffset=smiData.RigidTransform(7).translation  TranslationROffset=0  TranslationROffsetUnits=m  TranslationZOffset=0  TranslationZOffsetUnits=m  TranslationThetaOffset=0  TranslationThetaOffsetUnits=deg  RotationMethod=ArbitraryAxis  RotationAngleUnits=rad  RotationStandardAxis=+Z  RotationAngle=smiData.RigidTransform(7).angle  RotationArbitraryAxis=smiData.RigidTransform(7).axis  FollAlignAxisA=+X  BaseAlignAxisA=+Y  FollAlignAxisB=+Y  BaseAlignAxisB=+Z  RotationSequenceAxes=FollowerAxes  RotationSequence=XYX  RotationSequenceAngles=[0 0 0]  RotationSequenceAnglesUnits=deg  RotationMatrix=[1 0 0; 0 1 0; 0 0 1]
  F : PMIOPort  Port=1  Side=Right
  connections:
  Solid/RConn1 -- ReferenceFrame/RConn1 -- Transform/LConn1
  Transform/RConn1 -- F/RConn1

== system X001_AL5D_Assemby_RR_013/REAL PLANT/Encoder Error ==
  PS Add : fl_lib/Physical Signals/Functions/PS Add
  PS Constant : fl_lib/Physical Signals/Sources/PS Constant  constant=REE
  PS Gain : fl_lib/Physical Signals/Functions/PS Gain  gain=-1
  q_out : PMIOPort  Port=1  Side=Right
  q_in : PMIOPort  Port=2  Side=Left
  connections:
  PS Constant/RConn1 -- PS Add/LConn1
  q_out/RConn1 -- PS Add/RConn1
  q_in/RConn1 -- PS Gain/LConn1
  PS Gain/RConn1 -- PS Add/LConn2

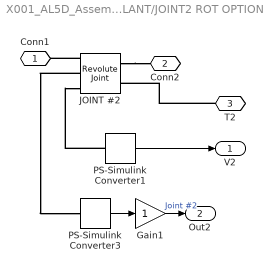
== system X001_AL5D_Assemby_RR_013/REAL PLANT/JOINT2 ROT OPTION ==
  Gain1 : Gain
  "JOINT #2 " : sm_lib/Joints/Revolute Joint  SenseConstraintForce=off  SenseConstraintForceX=off  SenseConstraintForceY=off  SenseConstraintForceZ=off  SenseConstraintTorque=off  SenseConstraintTorqueX=off  SenseConstraintTorqueY=off  SenseConstraintTorqueZ=off  SenseTotalForce=off  SenseTotalForceX=off  SenseTotalForceY=off  SenseTotalForceZ=off  SenseTotalTorque=off  SenseTotalTorqueX=off  SenseTotalTorqueY=off  SenseTotalTorqueZ=off  CompositeWrenchDir=FollowerOnBase  CompositeWrenchFrame=BaseFrame  EquilibriumPosition=0  EquilibriumPositionUnits=rad  SpringStiffness=JSS  SpringStiffnessUnits=m*N/rad  DampingCoefficient=JDC  DampingCoefficientUnits=m*s*N/rad  TorqueActuationMode=InputTorque  MotionActuationMode=ComputedMotion  SensePosition=on  SenseVelocity=on  SenseAcceleration=off  SenseTorqueForce=off  PositionTargetSpecify=off  PositionTargetPriority=Low  PositionTargetValue=45  PositionTargetValueUnits=deg  VelocityTargetSpecify=off  VelocityTargetPriority=High  VelocityTargetValue=0  VelocityTargetValueUnits=deg/s
  PS-Simulink Converter1 : nesl_utility/PS-Simulink Converter  PhysicalDomain=network_engine_domain  SubClassName=ps_output  LeftPortType=input  RightPortType=output  PseudoPeriodic=off  Frequencies=[]  Unit=rad/s  AffineConversion=off
  PS-Simulink Converter3 : nesl_utility/PS-Simulink Converter  PhysicalDomain=network_engine_domain  SubClassName=ps_output  LeftPortType=input  RightPortType=output  PseudoPeriodic=off  Frequencies=[]  Unit=rad  AffineConversion=off
  Conn1 : PMIOPort  Port=1  Side=Left
  Conn2 : PMIOPort  Port=2  Side=Right
  T2 : PMIOPort  Port=3  Side=Left
  V2 : Outport
  Out2 : Outport  Port=2
  wires:
  Gain1/1 -> Out2/1  "Joint #2"
  PS-Simulink Converter3/1 -> Gain1/1
  PS-Simulink Converter1/1 -> V2/1
  connections:
  "JOINT #2 "/RConn1 -- Conn1/RConn1
  "JOINT #2 "/LConn1 -- Conn2/RConn1
  T2/RConn1 -- "JOINT #2 "/LConn2
  "JOINT #2 "/RConn2 -- PS-Simulink Converter3/LConn1
  PS-Simulink Converter1/LConn1 -- "JOINT #2 "/RConn3

== system X001_AL5D_Assemby_RR_013/REAL PLANT/MID-ARM ==
  ReferenceFrame : sm_lib/Frames and Transforms/Reference Frame
  Solid : sm_lib/Body Elements/Solid  InertiaType=Custom  Mass=smiData.Solid(3).mass  MassUnits=kg  CenterOfMass=smiData.Solid(3).CoM  CenterOfMassUnits=mm  MomentsOfInertia=smiData.Solid(3).MoI  MomentsOfInertiaUnits=kg*mm^2  ProductsOfInertia=smiData.Solid(3).PoI  ProductsOfInertiaUnits=kg*mm^2  DensityBased=on  Density=1000  DensityUnits=kg/(m^3)  DoExposeReferenceFrame=on  SerializedFrames=<Frames/>  GraphicType=FromGeometry  MarkerShape=Sphere  MarkerSize=10  GraphicVisPropType=SimpleVisualProperties  GraphicDiffuseColor=smiData.Solid(3).color  GraphicSpecularColor=[0.5 0.5 0.5 1.0]  GraphicAmbientColor=[0.15 0.15 0.15 1.0]  GraphicEmissiveColor=[0.0 0.0 0.0 1.0]  GraphicShininess=75  GraphicOpacity=smiData.Solid(3).opacity  GeometryShape=FromFile  RectangleSize=[1 1]  RectangleSizeUnits=m  BrickDimensions=[1 1 1]  BrickDimensionUnits=m  CylinderRadius=1  CylinderRadiusUnits=m  CylinderLength=1  CylinderLengthUnits=m  SphereRadius=1  SphereRadiusUnits=m  EllipsoidRadii=[1 1 1]  EllipsoidRadiiUnits=m  ExtrusionCrossSection=[1 1; -1 1; -1 -1; 1 -1]  ExtrusionCrossSectionUnits=m  ExtrusionLength=1  ExtrusionLengthUnits=m  PolygonNumSides=3  PolygonOuterRadius=1  PolygonOuterRadiusUnits=m  ExtGeomFileType=STEP  ExtGeomFileName=003_Arm1_Subassy_Default_sldprt.STEP  ExtGeomFileUnits=m  RevolutionCrossSection=[1 1; 1 -1; 2 -1; 2 1]  RevolutionCrossSectionUnits=m  RevolutionExtent=Full  RevolutionAngle=180  RevolutionAngleUnits=deg
  Transform : sm_lib/Frames and Transforms/Rigid Transform  TranslationMethod=Cartesian  TranslationLengthUnit=mm  TranslationStandardAxis=+Z  TranslationStandardOffset=0  TranslationCartesianOffset=smiData.RigidTransform(4).translation  TranslationROffset=0  TranslationROffsetUnits=m  TranslationZOffset=0  TranslationZOffsetUnits=m  TranslationThetaOffset=0  TranslationThetaOffsetUnits=deg  RotationMethod=ArbitraryAxis  RotationAngleUnits=rad  RotationStandardAxis=+Z  RotationAngle=smiData.RigidTransform(4).angle  RotationArbitraryAxis=smiData.RigidTransform(4).axis  FollAlignAxisA=+X  BaseAlignAxisA=+Y  FollAlignAxisB=+Y  BaseAlignAxisB=+Z  RotationSequenceAxes=FollowerAxes  RotationSequence=XYX  RotationSequenceAngles=[0 0 0]  RotationSequenceAnglesUnits=deg  RotationMatrix=[1 0 0; 0 1 0; 0 0 1]
  Transform1 : sm_lib/Frames and Transforms/Rigid Transform  TranslationMethod=Cartesian  TranslationLengthUnit=mm  TranslationStandardAxis=+Z  TranslationStandardOffset=0  TranslationCartesianOffset=smiData.RigidTransform(8).translation  TranslationROffset=0  TranslationROffsetUnits=m  TranslationZOffset=0  TranslationZOffsetUnits=m  TranslationThetaOffset=0  TranslationThetaOffsetUnits=deg  RotationMethod=ArbitraryAxis  RotationAngleUnits=rad  RotationStandardAxis=+Z  RotationAngle=smiData.RigidTransform(8).angle  RotationArbitraryAxis=smiData.RigidTransform(8).axis  FollAlignAxisA=+X  BaseAlignAxisA=+Y  FollAlignAxisB=+Y  BaseAlignAxisB=+Z  RotationSequenceAxes=FollowerAxes  RotationSequence=XYX  RotationSequenceAngles=[0 0 0]  RotationSequenceAnglesUnits=deg  RotationMatrix=[1 0 0; 0 1 0; 0 0 1]
  F1 : PMIOPort  Port=1  Side=Right
  F : PMIOPort  Port=2  Side=Left
  connections:
  Solid/RConn1 -- ReferenceFrame/RConn1 -- Transform/LConn1 -- Transform1/LConn1
  Transform/RConn1 -- F/RConn1
  F1/RConn1 -- Transform1/RConn1

== system X001_AL5D_Assemby_RR_013/COLLISION SIMULATOR/Spring-Damper Contact/Enabled Subsystem ==
  In1 : Inport
  Enable : EnablePort
  Out1 : Outport
  wires:
  In1/1 -> Out1/1

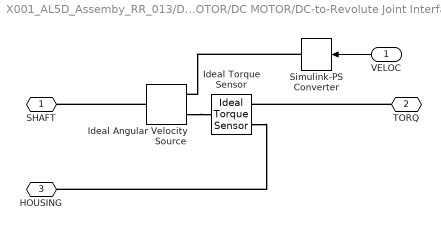
== system X001_AL5D_Assemby_RR_013/DC MOTOR/DC MOTOR/DC-to-Revolute Joint Interface ==
  VELOC : Inport
  Ideal Angular Velocity Source : fl_lib/Mechanical/Mechanical Sources/Ideal Angular Velocity Source
  Ideal Torque Sensor : fl_lib/Mechanical/Mechanical Sensors/Ideal Torque Sensor
  Simulink-PS Converter : nesl_utility/Simulink-PS Converter  PhysicalDomain=network_engine_domain  SubClassName=ps_input  LeftPortType=input  RightPortType=output  PseudoPeriodic=off  Frequencies=[]  NoiseDistribution=none  NoiseParameters=[]  Unit=deg/s  AffineConversion=off  InputFiltering=on  SimscapeFilterOrder=1  InputFilterTimeConstant=0.001  UdotUserProvided=1
  SHAFT : PMIOPort  Port=1  Side=Left
  TORQ : PMIOPort  Port=2  Side=Right
  HOUSING : PMIOPort  Port=3  Side=Left
  wires:
  VELOC/1 -> Simulink-PS Converter/1
  connections:
  TORQ/RConn1 -- Ideal Torque Sensor/RConn2
  Ideal Torque Sensor/RConn1 -- HOUSING/RConn1
  Simulink-PS Converter/RConn1 -- Ideal Angular Velocity Source/RConn1
  Ideal Angular Velocity Source/RConn2 -- Ideal Torque Sensor/LConn1
  Ideal Angular Velocity Source/LConn1 -- SHAFT/RConn1

== system X001_AL5D_Assemby_RR_013/DC MOTOR/DC MOTOR/SL2Vbrk ==
  Signal : Inport
  Electrical Reference1 : fl_lib/Electrical/Electrical Elements/Electrical Reference
  Simulink to Physical Signal1 : nesl_utility/Simulink-PS Converter  PhysicalDomain=network_engine_domain  SubClassName=ps_input  LeftPortType=input  RightPortType=output  PseudoPeriodic=off  Frequencies=[]  NoiseDistribution=none  NoiseParameters=[]  Unit=V  AffineConversion=off  InputFiltering=off  SimscapeFilterOrder=1  InputFilterTimeConstant=.001  UdotUserProvided=0
  Voltage Source : fl_lib/Electrical/Electrical Sources/Controlled Voltage Source
  Volts : PMIOPort  Tag=PMCPort  Port=1  Side=Right
  wires:
  Signal/1 -> Simulink to Physical Signal1/1
  connections:
  Electrical Reference1/LConn1 -- Voltage Source/RConn2
  Simulink to Physical Signal1/RConn1 -- Voltage Source/RConn1
  Voltage Source/LConn1 -- Volts/RConn1

== system X001_AL5D_Assemby_RR_013/DC MOTOR/DC MOTOR/SL2Vduty ==
  Signal : Inport
  Electrical Reference1 : fl_lib/Electrical/Electrical Elements/Electrical Reference
  Simulink to Physical Signal1 : nesl_utility/Simulink-PS Converter  PhysicalDomain=network_engine_domain  SubClassName=ps_input  LeftPortType=input  RightPortType=output  PseudoPeriodic=off  Frequencies=[]  NoiseDistribution=none  NoiseParameters=[]  Unit=V  AffineConversion=off  InputFiltering=off  SimscapeFilterOrder=1  InputFilterTimeConstant=.001  UdotUserProvided=0
  Voltage Source : fl_lib/Electrical/Electrical Sources/Controlled Voltage Source
  Volts : PMIOPort  Tag=PMCPort  Port=1  Side=Right
  wires:
  Signal/1 -> Simulink to Physical Signal1/1
  connections:
  Electrical Reference1/LConn1 -- Voltage Source/RConn2
  Simulink to Physical Signal1/RConn1 -- Voltage Source/RConn1
  Voltage Source/LConn1 -- Volts/RConn1

== system X001_AL5D_Assemby_RR_013/DC MOTOR/DC MOTOR/SL2Vrev ==
  Signal : Inport
  Electrical Reference1 : fl_lib/Electrical/Electrical Elements/Electrical Reference
  Simulink to Physical Signal1 : nesl_utility/Simulink-PS Converter  PhysicalDomain=network_engine_domain  SubClassName=ps_input  LeftPortType=input  RightPortType=output  PseudoPeriodic=off  Frequencies=[]  NoiseDistribution=none  NoiseParameters=[]  Unit=V  AffineConversion=off  InputFiltering=off  SimscapeFilterOrder=1  InputFilterTimeConstant=.001  UdotUserProvided=0
  Voltage Source : fl_lib/Electrical/Electrical Sources/Controlled Voltage Source
  Volts : PMIOPort  Tag=PMCPort  Port=1  Side=Right
  wires:
  Signal/1 -> Simulink to Physical Signal1/1
  connections:
  Voltage Source/LConn1 -- Volts/RConn1
  Simulink to Physical Signal1/RConn1 -- Voltage Source/RConn1
  Electrical Reference1/LConn1 -- Voltage Source/RConn2

== system X001_AL5D_Assemby_RR_013/INVERSE  ESTIMATED PLANT (DOB)/Inverse Estimated Plant/BASE ==
  ReferenceFrame : sm_lib/Frames and Transforms/Reference Frame
  Solid : sm_lib/Body Elements/Solid  InertiaType=Custom  Mass=smiData.Solid(2).mass  MassUnits=kg  CenterOfMass=smiData.Solid(2).CoM  CenterOfMassUnits=mm  MomentsOfInertia=smiData.Solid(2).MoI  MomentsOfInertiaUnits=kg*mm^2  ProductsOfInertia=smiData.Solid(2).PoI  ProductsOfInertiaUnits=kg*mm^2  DensityBased=on  Density=1000  DensityUnits=kg/(m^3)  DoExposeReferenceFrame=on  SerializedFrames=<Frames/>  GraphicType=FromGeometry  MarkerShape=Sphere  MarkerSize=10  GraphicVisPropType=SimpleVisualProperties  GraphicDiffuseColor=smiData.Solid(2).color  GraphicSpecularColor=[0.5 0.5 0.5 1.0]  GraphicAmbientColor=[0.15 0.15 0.15 1.0]  GraphicEmissiveColor=[0.0 0.0 0.0 1.0]  GraphicShininess=75  GraphicOpacity=smiData.Solid(2).opacity  GeometryShape=FromFile  RectangleSize=[1 1]  RectangleSizeUnits=m  BrickDimensions=[1 1 1]  BrickDimensionUnits=m  CylinderRadius=1  CylinderRadiusUnits=m  CylinderLength=1  CylinderLengthUnits=m  SphereRadius=1  SphereRadiusUnits=m  EllipsoidRadii=[1 1 1]  EllipsoidRadiiUnits=m  ExtrusionCrossSection=[1 1; -1 1; -1 -1; 1 -1]  ExtrusionCrossSectionUnits=m  ExtrusionLength=1  ExtrusionLengthUnits=m  PolygonNumSides=3  PolygonOuterRadius=1  PolygonOuterRadiusUnits=m  ExtGeomFileType=STEP  ExtGeomFileName=X001_AL5D_Base_Subassy_Default_sldprt.STEP  ExtGeomFileUnits=m  RevolutionCrossSection=[1 1; 1 -1; 2 -1; 2 1]  RevolutionCrossSectionUnits=m  RevolutionExtent=Full  RevolutionAngle=180  RevolutionAngleUnits=deg
  Transform : sm_lib/Frames and Transforms/Rigid Transform  TranslationMethod=Cartesian  TranslationLengthUnit=mm  TranslationStandardAxis=+Z  TranslationStandardOffset=0  TranslationCartesianOffset=smiData.RigidTransform(1).translation  TranslationROffset=0  TranslationROffsetUnits=m  TranslationZOffset=0  TranslationZOffsetUnits=m  TranslationThetaOffset=0  TranslationThetaOffsetUnits=deg  RotationMethod=ArbitraryAxis  RotationAngleUnits=rad  RotationStandardAxis=+Z  RotationAngle=smiData.RigidTransform(1).angle  RotationArbitraryAxis=smiData.RigidTransform(1).axis  FollAlignAxisA=+X  BaseAlignAxisA=+Y  FollAlignAxisB=+Y  BaseAlignAxisB=+Z  RotationSequenceAxes=FollowerAxes  RotationSequence=XYX  RotationSequenceAngles=[0 0 0]  RotationSequenceAnglesUnits=deg  RotationMatrix=[1 0 0; 0 1 0; 0 0 1]
  Transform1 : sm_lib/Frames and Transforms/Rigid Transform  TranslationMethod=Cartesian  TranslationLengthUnit=mm  TranslationStandardAxis=+Z  TranslationStandardOffset=0  TranslationCartesianOffset=smiData.RigidTransform(3).translation  TranslationROffset=0  TranslationROffsetUnits=m  TranslationZOffset=0  TranslationZOffsetUnits=m  TranslationThetaOffset=0  TranslationThetaOffsetUnits=deg  RotationMethod=ArbitraryAxis  RotationAngleUnits=rad  RotationStandardAxis=+Z  RotationAngle=smiData.RigidTransform(3).angle  RotationArbitraryAxis=smiData.RigidTransform(3).axis  FollAlignAxisA=+X  BaseAlignAxisA=+Y  FollAlignAxisB=+Y  BaseAlignAxisB=+Z  RotationSequenceAxes=FollowerAxes  RotationSequence=XYX  RotationSequenceAngles=[0 0 0]  RotationSequenceAnglesUnits=deg  RotationMatrix=[1 0 0; 0 1 0; 0 0 1]
  F : PMIOPort  Port=1  Side=Left
  F1 : PMIOPort  Port=2  Side=Right
  connections:
  Solid/RConn1 -- ReferenceFrame/RConn1 -- Transform/LConn1 -- Transform1/LConn1
  F1/RConn1 -- Transform1/RConn1
  F/RConn1 -- Transform/RConn1

== system X001_AL5D_Assemby_RR_013/INVERSE  ESTIMATED PLANT (DOB)/Inverse Estimated Plant/END EFFECTOR ==
  ReferenceFrame : sm_lib/Frames and Transforms/Reference Frame
  Solid : sm_lib/Body Elements/Solid  InertiaType=Custom  Mass=smiData.Solid(1).mass  MassUnits=kg  CenterOfMass=smiData.Solid(1).CoM  CenterOfMassUnits=mm  MomentsOfInertia=smiData.Solid(1).MoI  MomentsOfInertiaUnits=kg*mm^2  ProductsOfInertia=smiData.Solid(1).PoI  ProductsOfInertiaUnits=kg*mm^2  DensityBased=on  Density=1000  DensityUnits=kg/(m^3)  DoExposeReferenceFrame=on  SerializedFrames=<Frames/>  GraphicType=FromGeometry  MarkerShape=Sphere  MarkerSize=10  GraphicVisPropType=SimpleVisualProperties  GraphicDiffuseColor=smiData.Solid(1).color  GraphicSpecularColor=[0.5 0.5 0.5 1.0]  GraphicAmbientColor=[0.15 0.15 0.15 1.0]  GraphicEmissiveColor=[0.0 0.0 0.0 1.0]  GraphicShininess=75  GraphicOpacity=smiData.Solid(1).opacity  GeometryShape=FromFile  RectangleSize=[1 1]  RectangleSizeUnits=m  BrickDimensions=[1 1 1]  BrickDimensionUnits=m  CylinderRadius=1  CylinderRadiusUnits=m  CylinderLength=1  CylinderLengthUnits=m  SphereRadius=1  SphereRadiusUnits=m  EllipsoidRadii=[1 1 1]  EllipsoidRadiiUnits=m  ExtrusionCrossSection=[1 1; -1 1; -1 -1; 1 -1]  ExtrusionCrossSectionUnits=m  ExtrusionLength=1  ExtrusionLengthUnits=m  PolygonNumSides=3  PolygonOuterRadius=1  PolygonOuterRadiusUnits=m  ExtGeomFileType=STEP  ExtGeomFileName=End_effector_subassy_Default_sldprt.STEP  ExtGeomFileUnits=m  RevolutionCrossSection=[1 1; 1 -1; 2 -1; 2 1]  RevolutionCrossSectionUnits=m  RevolutionExtent=Full  RevolutionAngle=180  RevolutionAngleUnits=deg
  Transform : sm_lib/Frames and Transforms/Rigid Transform  TranslationMethod=Cartesian  TranslationLengthUnit=mm  TranslationStandardAxis=+Z  TranslationStandardOffset=0  TranslationCartesianOffset=smiData.RigidTransform(7).translation  TranslationROffset=0  TranslationROffsetUnits=m  TranslationZOffset=0  TranslationZOffsetUnits=m  TranslationThetaOffset=0  TranslationThetaOffsetUnits=deg  RotationMethod=ArbitraryAxis  RotationAngleUnits=rad  RotationStandardAxis=+Z  RotationAngle=smiData.RigidTransform(7).angle  RotationArbitraryAxis=smiData.RigidTransform(7).axis  FollAlignAxisA=+X  BaseAlignAxisA=+Y  FollAlignAxisB=+Y  BaseAlignAxisB=+Z  RotationSequenceAxes=FollowerAxes  RotationSequence=XYX  RotationSequenceAngles=[0 0 0]  RotationSequenceAnglesUnits=deg  RotationMatrix=[1 0 0; 0 1 0; 0 0 1]
  F : PMIOPort  Port=1  Side=Right
  connections:
  Solid/RConn1 -- ReferenceFrame/RConn1 -- Transform/LConn1
  Transform/RConn1 -- F/RConn1
